simulink model "projeto_fixedstepdiscrete"  (R2015a)
settings: Solver=FixedStepDiscrete  SolverMode=SingleTasking  StartTime=0.0  StopTime=inf  RelTol=1e-3
libraries: dsparch4 x17, dspvision x14, commchan3 x1, dspsnks4 x1
settings Model: SimulationMode=accelerator  Creator=aluno  LastModifiedBy=aluno
settings DataIOCC: SaveOutput=off  SignalLogging=off  SaveTime=off
settings DebuggingCC: AlgebraicLoopMsg=error  SingleTaskRateTransMsg=error

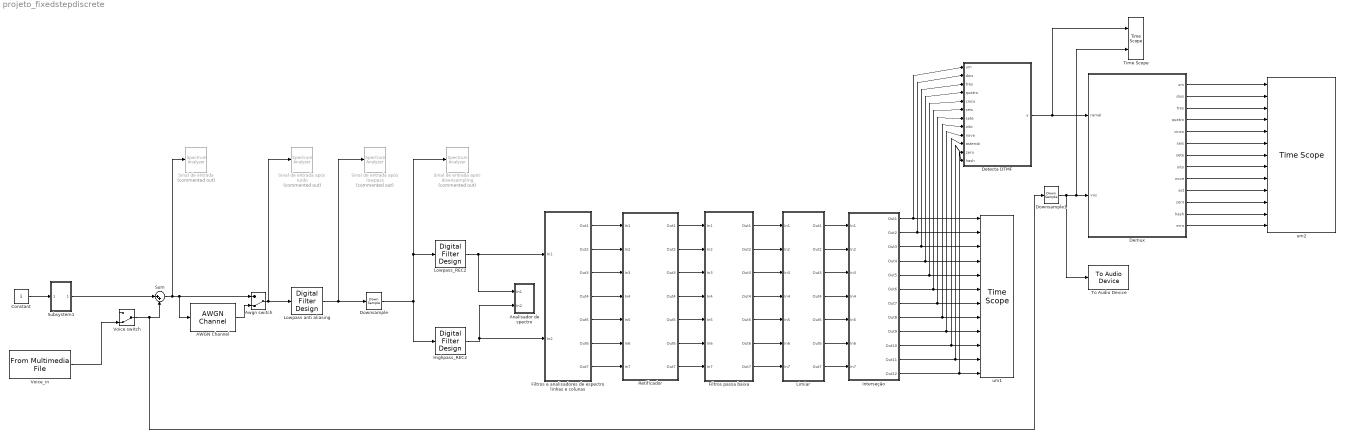
== system projeto_fixedstepdiscrete ==
  AWGN Channel : commchan3/AWGN Channel  InputProcessing=Columns as channels (frame based)  seed=67  noiseMode="Signal to noise ratio  (SNR)"  EbNodB=30  EsNodB=10  SNRdB=5  bitsPerSym=1  Ps=1  Tsym=1  variance=1
  Analisador de spectro : Subsystem
  Awgn switch : ManualSwitch  CurrentSetting=0
  Constant : Constant
  Demux : MATLAB Function  TreatAsAtomicUnit=on
  Detecta DTMF : MATLAB Function  TreatAsAtomicUnit=on
  Downsample : DownSample  N=11  RateOptions=Allow multirate processing
  Downsample1 : DownSample  N=11  RateOptions=Allow multirate processing
  Filtros e analisadores de espectro linhas e colunas : Subsystem
  Filtros passa baixa : Subsystem
  "Highpass_REC2 " : dsparch4/Digital Filter Design  mwdsp_browser_bugfix_var=off
  Interseção : Subsystem
  Limiar : Subsystem
  Lowpass anti aliasing : dsparch4/Digital Filter Design  mwdsp_browser_bugfix_var=off
  Lowpass_REC2 : dsparch4/Digital Filter Design  mwdsp_browser_bugfix_var=off
  Retificador : Subsystem
  "Sinal de entrada " : SpectrumAnalyzer  Commented=on
  "Sinal de entrada após downsampling " : SpectrumAnalyzer  Commented=on
  "Sinal de entrada após lowpass " : SpectrumAnalyzer  Commented=on
  "Sinal de entrada após ruído " : SpectrumAnalyzer  Commented=on
  Subsystem1 : Subsystem
  Sum : Sum  Inputs=|++
  Time Scope : TimeScope  DefaultConfigurationName=spbscopes.TimeScopeBlockCfg  NumInputPorts=2
  To Audio Device : dspsnks4/To Audio Device  deviceName=Default  inheritSampleRate=on  sampleRate=44100  deviceDatatype=Determine from input data type  autoBufferSize=on  bufferSize=4096  queueDuration=1.0  defaultOutputChannelMapping=on  outputChannelMapping=1:2  outputNumUnderrunSamples=off
  Voice switch : ManualSwitch  CurrentSetting=0
  "Voice_in " : dspvision/From Multimedia File  inputFilename=./Projeto_Final_PSD/Voice/voice.wav  loop=on  numPlays=inf  outputStreams=Audio only  videoDataType=single  audioDataType=double  inheritSampleTime=on  userDefinedSampleTime=1/30  noAudioOutput=off  isIntensityVideo=off  fourcc=RGB  colorVideoFormat=Separate color signals  outputEOF=off  dataOrg=Column-major  audioFrameSize=spc  computeAudioFrameSize=off  outSamplingMode=Sample based
  um1 : TimeScope  DefaultConfigurationName=spbscopes.TimeScopeBlockCfg  NumInputPorts=12
  um2 : TimeScope  DefaultConfigurationName=spbscopes.TimeScopeBlockCfg  NumInputPorts=13
  wires:
  "Voice_in "/1 -> Voice switch/2
  AWGN Channel/1 -> Awgn switch/2
  Awgn switch/1 -> Lowpass anti aliasing/1, "Sinal de entrada após ruído "/1
  Sum/1 -> "Sinal de entrada "/1, Awgn switch/1, AWGN Channel/1
  Lowpass_REC2/1 -> Analisador de spectro/1(In1), Filtros e analisadores de espectro linhas e colunas/1(In1)
  "Highpass_REC2 "/1 -> Analisador de spectro/2(In2), Filtros e analisadores de espectro linhas e colunas/2(In2)
  Downsample/1 -> "Highpass_REC2 "/1, Lowpass_REC2/1, "Sinal de entrada após downsampling "/1
  Filtros e analisadores de espectro linhas e colunas/1(Out1) -> Retificador/1(In1)
  Filtros e analisadores de espectro linhas e colunas/2(Out2) -> Retificador/2(In2)
  Filtros e analisadores de espectro linhas e colunas/3(Out3) -> Retificador/3(In3)
  Filtros e analisadores de espectro linhas e colunas/4(Out4) -> Retificador/4(In4)
  Filtros e analisadores de espectro linhas e colunas/5(Out5) -> Retificador/5(In5)
  Filtros e analisadores de espectro linhas e colunas/6(Out6) -> Retificador/6(In6)
  Filtros e analisadores de espectro linhas e colunas/7(Out7) -> Retificador/7(In7)
  Constant/1 -> Subsystem1/1(In1)
  Subsystem1/1(Out1) -> Sum/1
  Lowpass anti aliasing/1 -> Downsample/1, "Sinal de entrada após lowpass "/1
  Retificador/1(Out1) -> Filtros passa baixa/1(In1)
  Retificador/2(Out2) -> Filtros passa baixa/2(In2)
  Retificador/3(Out3) -> Filtros passa baixa/3(In3)
  Retificador/4(Out4) -> Filtros passa baixa/4(In4)
  Retificador/5(Out5) -> Filtros passa baixa/5(In5)
  Retificador/6(Out6) -> Filtros passa baixa/6(In6)
  Retificador/7(Out7) -> Filtros passa baixa/7(In7)
  Filtros passa baixa/1(Out1) -> Limiar/1(In1)
  Filtros passa baixa/2(Out2) -> Limiar/2(In2)
  Filtros passa baixa/3(Out3) -> Limiar/3(In3)
  Filtros passa baixa/4(Out4) -> Limiar/4(In4)
  Filtros passa baixa/5(Out5) -> Limiar/5(In5)
  Filtros passa baixa/6(Out6) -> Limiar/6(In6)
  Filtros passa baixa/7(Out7) -> Limiar/7(In7)
  Limiar/1(Out1) -> Interseção/1(In1)
  Limiar/2(Out2) -> Interseção/2(In2)
  Limiar/3(Out3) -> Interseção/3(In3)
  Limiar/4(Out4) -> Interseção/4(In4)
  Limiar/5(Out5) -> Interseção/5(In5)
  Limiar/6(Out6) -> Interseção/6(In6)
  Limiar/7(Out7) -> Interseção/7(In7)
  Interseção/1(Out1) -> Detecta DTMF/1(um), um1/1
  Interseção/2(Out2) -> Detecta DTMF/2(dois), um1/2
  Interseção/3(Out3) -> Detecta DTMF/3(tres), um1/3
  Interseção/5(Out5) -> um1/5, Detecta DTMF/5(cinco)
  Interseção/6(Out6) -> um1/6, Detecta DTMF/6(seis)
  Interseção/7(Out7) -> Detecta DTMF/7(sete), um1/7
  Interseção/8(Out8) -> Detecta DTMF/8(oito), um1/8
  Interseção/9(Out9) -> Detecta DTMF/9(nove), um1/9
  Interseção/10(Out10) -> Detecta DTMF/10(asterisk), um1/10
  Interseção/11(Out11) -> Detecta DTMF/11(zero), um1/11
  Interseção/12(Out12) -> Detecta DTMF/12(hash), um1/12
  Interseção/4(Out4) -> Detecta DTMF/4(quatro), um1/4
  Demux/1(um) -> um2/1
  Demux/2(dois) -> um2/2
  Demux/3(tres) -> um2/3
  Demux/4(quatro) -> um2/4
  Demux/5(cinco) -> um2/5
  Demux/6(seis) -> um2/6
  Demux/7(sete) -> um2/7
  Demux/8(oito) -> um2/8
  Demux/9(nove) -> um2/9
  Demux/10(ast) -> um2/10
  Demux/11(zero) -> um2/11
  Demux/12(hash) -> um2/12
  Voice switch/1 -> Sum/2, Downsample1/1
  Demux/13(erro) -> um2/13
  Detecta DTMF/1(y) -> Demux/1(ramal), Time Scope/1
  Downsample1/1 -> To Audio Device/1, Time Scope/2, Demux/2(voz)

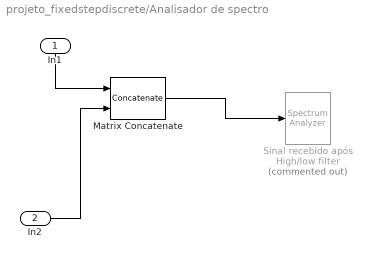
== system projeto_fixedstepdiscrete/Analisador de spectro ==
  In1 : Inport
  In2 : Inport  Port=2
  Matrix Concatenate : Concatenate  Mode=Multidimensional array  ConcatenateDimension=2
  Sinal recebido após High/low filter : SpectrumAnalyzer  Commented=on
  wires:
  In1/1 -> Matrix Concatenate/1
  In2/1 -> Matrix Concatenate/2
  Matrix Concatenate/1 -> Sinal recebido após High/low filter/1

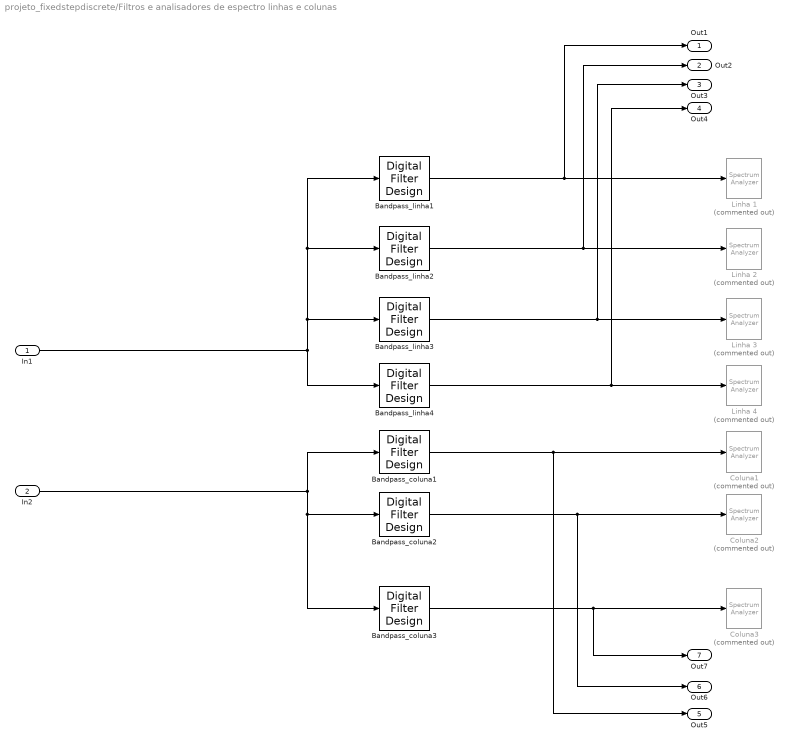
== system projeto_fixedstepdiscrete/Filtros e analisadores de espectro linhas e colunas ==
  In1 : Inport
  In2 : Inport  Port=2
  Bandpass_coluna1 : dsparch4/Digital Filter Design  mwdsp_browser_bugfix_var=off
  Bandpass_coluna2 : dsparch4/Digital Filter Design  mwdsp_browser_bugfix_var=off
  Bandpass_coluna3 : dsparch4/Digital Filter Design  mwdsp_browser_bugfix_var=off
  Bandpass_linha{1..4} (4 alike) : dsparch4/Digital Filter Design  mwdsp_browser_bugfix_var=off
  "Coluna1 " : SpectrumAnalyzer  Commented=on
  "Coluna2 " : SpectrumAnalyzer  Commented=on
  Coluna3 : SpectrumAnalyzer  Commented=on
  Linha {1..4} (4 alike) : SpectrumAnalyzer  Commented=on
  Out1 : Outport
  Out2 : Outport  Port=2
  Out3 : Outport  Port=3
  Out4 : Outport  Port=4
  Out5 : Outport  Port=5
  Out6 : Outport  Port=6
  Out7 : Outport  Port=7
  wires:
  In1/1 -> Bandpass_linha4/1, Bandpass_linha3/1, Bandpass_linha2/1, Bandpass_linha1/1
  In2/1 -> Bandpass_coluna1/1, Bandpass_coluna2/1, Bandpass_coluna3/1
  Bandpass_linha1/1 -> Out1/1, Linha 1/1
  Bandpass_linha4/1 -> Out4/1, Linha 4/1
  Bandpass_linha2/1 -> Out2/1, Linha 2/1
  Bandpass_coluna3/1 -> Out7/1, Coluna3/1
  Bandpass_coluna2/1 -> Out6/1, "Coluna2 "/1
  Bandpass_linha3/1 -> Out3/1, Linha 3/1
  Bandpass_coluna1/1 -> Out5/1, "Coluna1 "/1

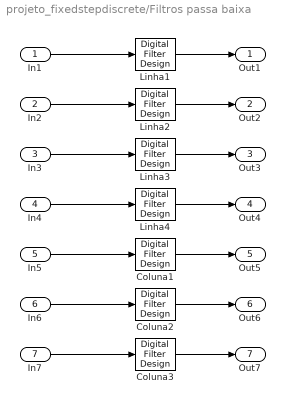
== system projeto_fixedstepdiscrete/Filtros passa baixa ==
  In1 : Inport
  In2 : Inport  Port=2
  In3 : Inport  Port=3
  In4 : Inport  Port=4
  In5 : Inport  Port=5
  In6 : Inport  Port=6
  In7 : Inport  Port=7
  Coluna1 : dsparch4/Digital Filter Design  mwdsp_browser_bugfix_var=off
  Coluna2 : dsparch4/Digital Filter Design  mwdsp_browser_bugfix_var=off
  Coluna3 : dsparch4/Digital Filter Design  mwdsp_browser_bugfix_var=off
  Linha{1..4} (4 alike) : dsparch4/Digital Filter Design  mwdsp_browser_bugfix_var=off
  Out1 : Outport
  Out2 : Outport  Port=2
  Out3 : Outport  Port=3
  Out4 : Outport  Port=4
  Out5 : Outport  Port=5
  Out6 : Outport  Port=6
  Out7 : Outport  Port=7
  wires:
  Linha2/1 -> Out2/1
  Coluna3/1 -> Out7/1
  Linha4/1 -> Out4/1
  Linha3/1 -> Out3/1
  In1/1 -> Linha1/1
  In2/1 -> Linha2/1
  In3/1 -> Linha3/1
  In4/1 -> Linha4/1
  In5/1 -> Coluna1/1
  In6/1 -> Coluna2/1
  In7/1 -> Coluna3/1
  Linha1/1 -> Out1/1
  Coluna1/1 -> Out5/1
  Coluna2/1 -> Out6/1

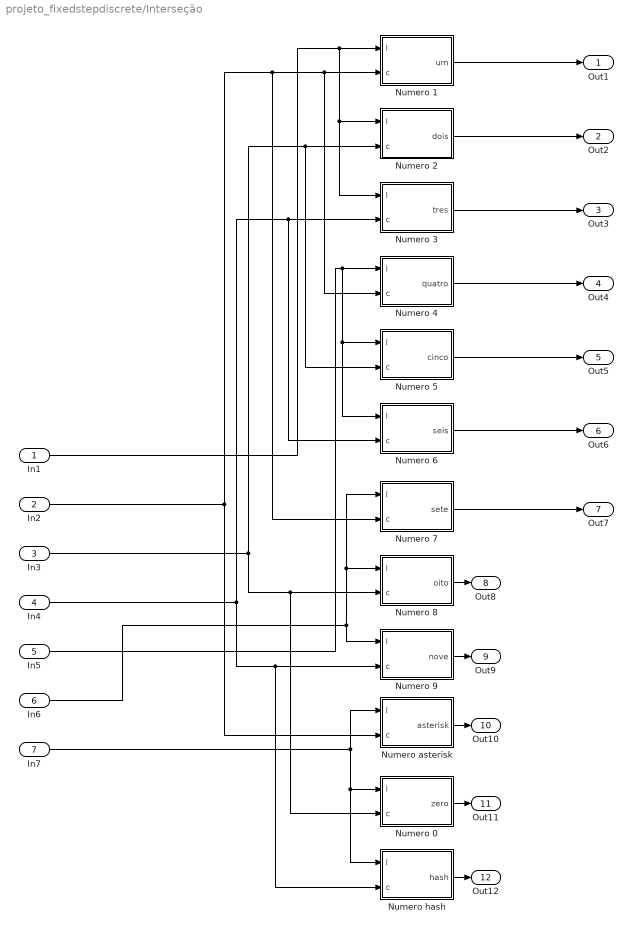
== system projeto_fixedstepdiscrete/Interseção ==
  In1 : Inport
  In2 : Inport  Port=2
  In3 : Inport  Port=3
  In4 : Inport  Port=4
  In5 : Inport  Port=5
  In6 : Inport  Port=6
  In7 : Inport  Port=7
  Numero 0 : MATLAB Function  TreatAsAtomicUnit=on
  Numero 1 : MATLAB Function  TreatAsAtomicUnit=on
  Numero 2 : MATLAB Function  TreatAsAtomicUnit=on
  Numero 3 : MATLAB Function  TreatAsAtomicUnit=on
  Numero 4 : MATLAB Function  TreatAsAtomicUnit=on
  Numero 5 : MATLAB Function  TreatAsAtomicUnit=on
  Numero 6 : MATLAB Function  TreatAsAtomicUnit=on
  Numero 7 : MATLAB Function  TreatAsAtomicUnit=on
  Numero 8 : MATLAB Function  TreatAsAtomicUnit=on
  Numero 9 : MATLAB Function  TreatAsAtomicUnit=on
  Numero asterisk : MATLAB Function  TreatAsAtomicUnit=on
  Numero hash : MATLAB Function  TreatAsAtomicUnit=on
  Out1 : Outport
  Out2 : Outport  Port=2
  Out3 : Outport  Port=3
  Out4 : Outport  Port=4
  Out5 : Outport  Port=5
  Out6 : Outport  Port=6
  Out7 : Outport  Port=7
  Out8 : Outport  Port=8
  Out9 : Outport  Port=9
  Out10 : Outport  Port=10
  Out11 : Outport  Port=11
  Out12 : Outport  Port=12
  wires:
  Numero 4/1(quatro) -> Out4/1
  Numero 9/1(nove) -> Out9/1
  In5/1 -> Numero 4/1(l), Numero 6/1(l), Numero 5/1(l)
  Numero 2/1(dois) -> Out2/1
  In1/1 -> Numero 3/1(l), Numero 2/1(l), Numero 1/1(l)
  Numero 5/1(cinco) -> Out5/1
  Numero 8/1(oito) -> Out8/1
  In3/1 -> Numero 0/2(c), Numero 8/2(c), Numero 5/2(c), Numero 2/2(c)
  In7/1 -> Numero hash/1(l), Numero 0/1(l), Numero asterisk/1(l)
  Numero 0/1(zero) -> Out11/1
  Numero hash/1(hash) -> Out12/1
  In6/1 -> Numero 7/1(l), Numero 8/1(l), Numero 9/1(l)
  Numero 7/1(sete) -> Out7/1
  Numero 6/1(seis) -> Out6/1
  Numero 3/1(tres) -> Out3/1
  In4/1 -> Numero hash/2(c), Numero 9/2(c), Numero 6/2(c), Numero 3/2(c)
  Numero asterisk/1(asterisk) -> Out10/1
  In2/1 -> Numero asterisk/2(c), Numero 7/2(c), Numero 4/2(c), Numero 1/2(c)
  Numero 1/1(um) -> Out1/1

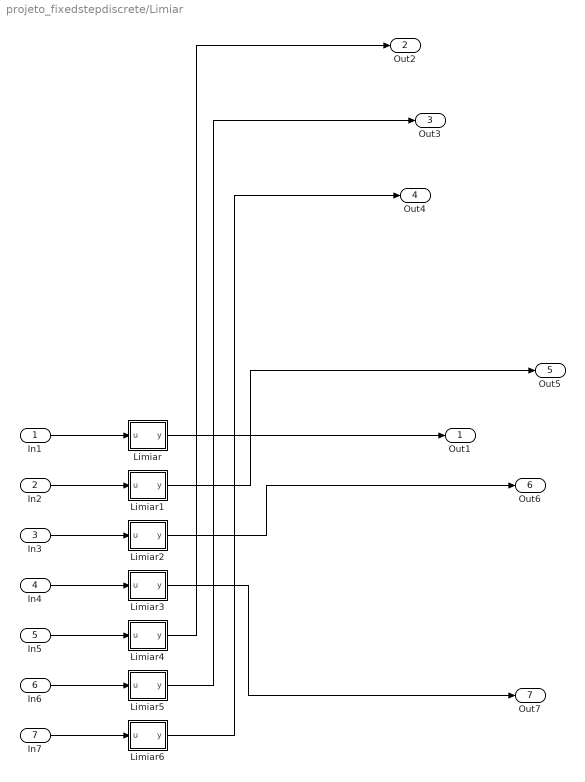
== system projeto_fixedstepdiscrete/Limiar ==
  In1 : Inport
  In2 : Inport  Port=2
  In3 : Inport  Port=3
  In4 : Inport  Port=4
  In5 : Inport  Port=5
  In6 : Inport  Port=6
  In7 : Inport  Port=7
  Limiar : MATLAB Function  TreatAsAtomicUnit=on
  Limiar1 : MATLAB Function  TreatAsAtomicUnit=on
  Limiar2 : MATLAB Function  TreatAsAtomicUnit=on
  Limiar3 : MATLAB Function  TreatAsAtomicUnit=on
  Limiar4 : MATLAB Function  TreatAsAtomicUnit=on
  Limiar5 : MATLAB Function  TreatAsAtomicUnit=on
  Limiar6 : MATLAB Function  TreatAsAtomicUnit=on
  Out1 : Outport
  Out2 : Outport  Port=2
  Out3 : Outport  Port=3
  Out4 : Outport  Port=4
  Out5 : Outport  Port=5
  Out6 : Outport  Port=6
  Out7 : Outport  Port=7
  wires:
  Limiar2/1(y) -> Out6/1
  Limiar4/1(y) -> Out2/1
  Limiar/1(y) -> Out1/1
  Limiar1/1(y) -> Out5/1
  In1/1 -> Limiar/1(u)
  In7/1 -> Limiar6/1(u)
  In6/1 -> Limiar5/1(u)
  In5/1 -> Limiar4/1(u)
  In3/1 -> Limiar2/1(u)
  In4/1 -> Limiar3/1(u)
  In2/1 -> Limiar1/1(u)
  Limiar6/1(y) -> Out4/1
  Limiar3/1(y) -> Out7/1
  Limiar5/1(y) -> Out3/1

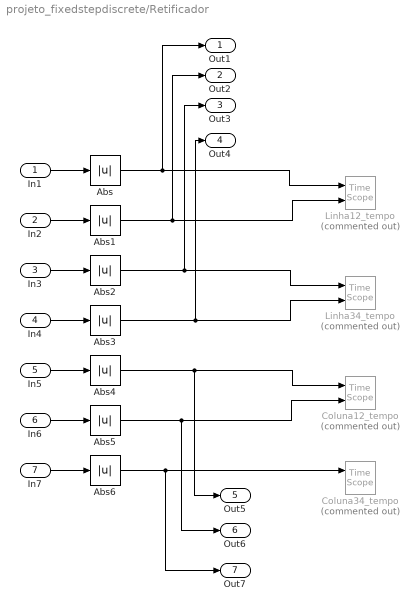
== system projeto_fixedstepdiscrete/Retificador ==
  In1 : Inport
  In2 : Inport  Port=2
  In3 : Inport  Port=3
  In4 : Inport  Port=4
  In5 : Inport  Port=5
  In6 : Inport  Port=6
  In7 : Inport  Port=7
  Abs{,1..6} (7 alike) : Abs
  Coluna12_tempo : TimeScope  Commented=on  DefaultConfigurationName=spbscopes.TimeScopeBlockCfg  NumInputPorts=2
  Coluna34_tempo : TimeScope  Commented=on  DefaultConfigurationName=spbscopes.TimeScopeBlockCfg  NumInputPorts=2
  "Linha12_tempo " : TimeScope  Commented=on  DefaultConfigurationName=spbscopes.TimeScopeBlockCfg  NumInputPorts=2
  Linha34_tempo : TimeScope  Commented=on  DefaultConfigurationName=spbscopes.TimeScopeBlockCfg  NumInputPorts=2
  Out1 : Outport
  Out2 : Outport  Port=2
  Out3 : Outport  Port=3
  Out4 : Outport  Port=4
  Out5 : Outport  Port=5
  Out6 : Outport  Port=6
  Out7 : Outport  Port=7
  wires:
  Abs6/1 -> Out7/1, Coluna34_tempo/1
  Abs5/1 -> Coluna12_tempo/2, Out6/1
  Abs4/1 -> Out5/1, Coluna12_tempo/1
  Abs2/1 -> Out3/1, Linha34_tempo/1
  Abs3/1 -> Out4/1, Linha34_tempo/2
  In6/1 -> Abs5/1
  In3/1 -> Abs2/1
  In4/1 -> Abs3/1
  In2/1 -> Abs1/1
  Abs1/1 -> Out2/1, "Linha12_tempo "/2
  In7/1 -> Abs6/1
  Abs/1 -> Out1/1, "Linha12_tempo "/1
  In5/1 -> Abs4/1
  In1/1 -> Abs/1

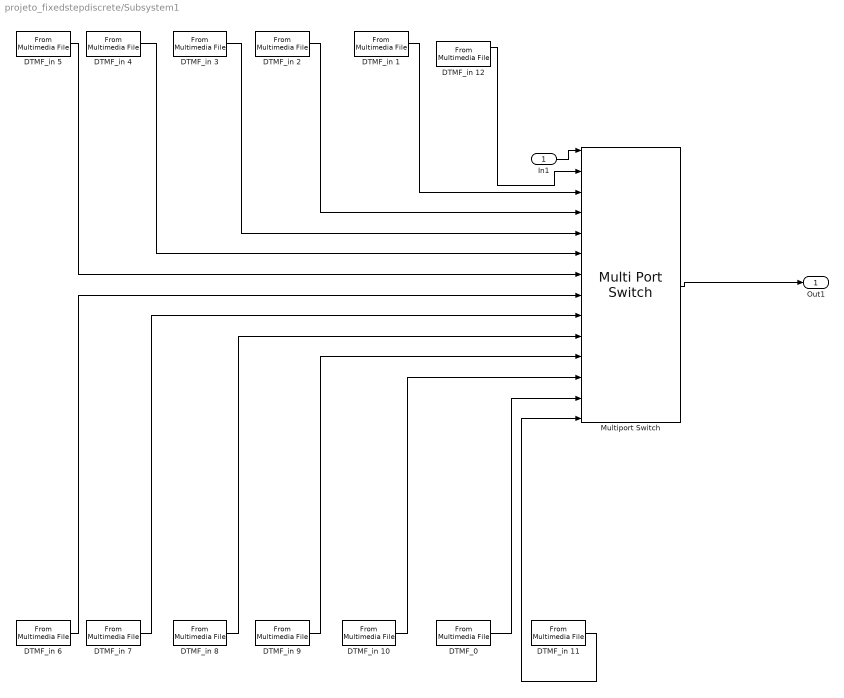
== system projeto_fixedstepdiscrete/Subsystem1 ==
  In1 : Inport
  "DTMF_0 " : dspvision/From Multimedia File  inputFilename=./Projeto_Final_PSD/Audios DTMF com Pausa/0-DTMF.wav  loop=on  numPlays=inf  outputStreams=Audio only  videoDataType=single  audioDataType=double  inheritSampleTime=on  userDefinedSampleTime=1/30  noAudioOutput=off  isIntensityVideo=off  fourcc=RGB  colorVideoFormat=Separate color signals  outputEOF=off  dataOrg=Column-major  audioFrameSize=spc  computeAudioFrameSize=off  outSamplingMode=Sample based
  DTMF_in 1 : dspvision/From Multimedia File  inputFilename=./Projeto_Final_PSD/Audios DTMF com Pausa/1-DTMF.wav  loop=on  numPlays=inf  outputStreams=Audio only  videoDataType=single  audioDataType=double  inheritSampleTime=on  userDefinedSampleTime=1/30  noAudioOutput=off  isIntensityVideo=off  fourcc=RGB  colorVideoFormat=Separate color signals  outputEOF=off  dataOrg=Column-major  audioFrameSize=spc  computeAudioFrameSize=off  outSamplingMode=Sample based
  DTMF_in 10 : dspvision/From Multimedia File  inputFilename=./Projeto_Final_PSD/Audios DTMF com Pausa/Asterisk.wav  loop=on  numPlays=inf  outputStreams=Audio only  videoDataType=single  audioDataType=double  inheritSampleTime=on  userDefinedSampleTime=1/30  noAudioOutput=off  isIntensityVideo=off  fourcc=RGB  colorVideoFormat=Separate color signals  outputEOF=off  dataOrg=Column-major  audioFrameSize=spc  computeAudioFrameSize=off  outSamplingMode=Sample based
  DTMF_in 11 : dspvision/From Multimedia File  inputFilename=./Projeto_Final_PSD/Audios DTMF com Pausa/Hash-DTMF.wav  loop=on  numPlays=inf  outputStreams=Audio only  videoDataType=single  audioDataType=double  inheritSampleTime=on  userDefinedSampleTime=1/30  noAudioOutput=off  isIntensityVideo=off  fourcc=RGB  colorVideoFormat=Separate color signals  outputEOF=off  dataOrg=Column-major  audioFrameSize=spc  computeAudioFrameSize=off  outSamplingMode=Sample based
  DTMF_in 12 : dspvision/From Multimedia File  inputFilename=./Projeto_Final_PSD/Audios DTMF com Pausa/Sequencia-DTMF.wav  loop=on  numPlays=inf  outputStreams=Audio only  videoDataType=single  audioDataType=double  inheritSampleTime=on  userDefinedSampleTime=1/30  noAudioOutput=off  isIntensityVideo=off  fourcc=RGB  colorVideoFormat=Separate color signals  outputEOF=on  dataOrg=Column-major  audioFrameSize=spc  computeAudioFrameSize=off  outSamplingMode=Sample based
  DTMF_in 2 : dspvision/From Multimedia File  inputFilename=./Projeto_Final_PSD/Audios DTMF com Pausa/2-DTMF.wav  loop=on  numPlays=inf  outputStreams=Audio only  videoDataType=single  audioDataType=double  inheritSampleTime=on  userDefinedSampleTime=1/30  noAudioOutput=off  isIntensityVideo=off  fourcc=RGB  colorVideoFormat=Separate color signals  outputEOF=off  dataOrg=Column-major  audioFrameSize=spc  computeAudioFrameSize=off  outSamplingMode=Sample based
  DTMF_in 3 : dspvision/From Multimedia File  inputFilename=./Projeto_Final_PSD/Audios DTMF com Pausa/3-DTMF.wav  loop=on  numPlays=inf  outputStreams=Audio only  videoDataType=single  audioDataType=double  inheritSampleTime=on  userDefinedSampleTime=1/30  noAudioOutput=off  isIntensityVideo=off  fourcc=RGB  colorVideoFormat=Separate color signals  outputEOF=off  dataOrg=Column-major  audioFrameSize=spc  computeAudioFrameSize=off  outSamplingMode=Sample based
  DTMF_in 4 : dspvision/From Multimedia File  inputFilename=./Projeto_Final_PSD/Audios DTMF com Pausa/4-DTMF.wav  loop=on  numPlays=inf  outputStreams=Audio only  videoDataType=single  audioDataType=double  inheritSampleTime=on  userDefinedSampleTime=1/30  noAudioOutput=off  isIntensityVideo=off  fourcc=RGB  colorVideoFormat=Separate color signals  outputEOF=off  dataOrg=Column-major  audioFrameSize=spc  computeAudioFrameSize=off  outSamplingMode=Sample based
  DTMF_in 5 : dspvision/From Multimedia File  inputFilename=./Projeto_Final_PSD/Audios DTMF com Pausa/5-DTMF.wav  loop=on  numPlays=inf  outputStreams=Audio only  videoDataType=single  audioDataType=double  inheritSampleTime=on  userDefinedSampleTime=1/30  noAudioOutput=off  isIntensityVideo=off  fourcc=RGB  colorVideoFormat=Separate color signals  outputEOF=off  dataOrg=Column-major  audioFrameSize=spc  computeAudioFrameSize=off  outSamplingMode=Sample based
  DTMF_in 6 : dspvision/From Multimedia File  inputFilename=./Projeto_Final_PSD/Audios DTMF com Pausa/6-DTMF.wav  loop=on  numPlays=inf  outputStreams=Audio only  videoDataType=single  audioDataType=double  inheritSampleTime=on  userDefinedSampleTime=1/30  noAudioOutput=off  isIntensityVideo=off  fourcc=RGB  colorVideoFormat=Separate color signals  outputEOF=off  dataOrg=Column-major  audioFrameSize=spc  computeAudioFrameSize=off  outSamplingMode=Sample based
  DTMF_in 7 : dspvision/From Multimedia File  inputFilename=./Projeto_Final_PSD/Audios DTMF com Pausa/7-DTMF.wav  loop=on  numPlays=inf  outputStreams=Audio only  videoDataType=single  audioDataType=double  inheritSampleTime=on  userDefinedSampleTime=1/30  noAudioOutput=off  isIntensityVideo=off  fourcc=RGB  colorVideoFormat=Separate color signals  outputEOF=off  dataOrg=Column-major  audioFrameSize=spc  computeAudioFrameSize=off  outSamplingMode=Sample based
  DTMF_in 8 : dspvision/From Multimedia File  inputFilename=./Projeto_Final_PSD/Audios DTMF com Pausa/8-DTMF.wav  loop=on  numPlays=inf  outputStreams=Audio only  videoDataType=single  audioDataType=double  inheritSampleTime=on  userDefinedSampleTime=1/30  noAudioOutput=off  isIntensityVideo=off  fourcc=RGB  colorVideoFormat=Separate color signals  outputEOF=off  dataOrg=Column-major  audioFrameSize=spc  computeAudioFrameSize=off  outSamplingMode=Sample based
  DTMF_in 9 : dspvision/From Multimedia File  inputFilename=./Projeto_Final_PSD/Audios DTMF com Pausa/9-DTMF.wav  loop=on  numPlays=inf  outputStreams=Audio only  videoDataType=single  audioDataType=double  inheritSampleTime=on  userDefinedSampleTime=1/30  noAudioOutput=off  isIntensityVideo=off  fourcc=RGB  colorVideoFormat=Separate color signals  outputEOF=off  dataOrg=Column-major  audioFrameSize=spc  computeAudioFrameSize=off  outSamplingMode=Sample based
  Multiport Switch : MultiPortSwitch  DataPortOrder=Specify indices  Inputs=12  DataPortIndices={0,1,2,3,4,5,6,7,8,9,10,11,12}
  Out1 : Outport
  wires:
  DTMF_in 7/1 -> Multiport Switch/9
  Multiport Switch/1 -> Out1/1
  DTMF_in 3/1 -> Multiport Switch/5
  DTMF_in 5/1 -> Multiport Switch/7
  DTMF_in 8/1 -> Multiport Switch/10
  In1/1 -> Multiport Switch/1
  DTMF_in 1/1 -> Multiport Switch/3
  DTMF_in 4/1 -> Multiport Switch/6
  DTMF_in 9/1 -> Multiport Switch/11
  DTMF_in 10/1 -> Multiport Switch/12
  DTMF_in 2/1 -> Multiport Switch/4
  DTMF_in 6/1 -> Multiport Switch/8
  DTMF_in 12/1 -> Multiport Switch/2
  "DTMF_0 "/1 -> Multiport Switch/13
  DTMF_in 11/1 -> Multiport Switch/14

== matlab function projeto_fixedstepdiscrete/Interseção/Numero 2 ==
  data: l input; dois output; c input

function dois = fcn(l,c)
%#codegen

if (l == 1 && c == 1) 
    u = 1;
else 
    u = 0;
end


dois = u;

== matlab function projeto_fixedstepdiscrete/Limiar/Limiar ==
  data: u input; y output

function y = fcn(u)
%#codegen

u = (u>0.2);

y = u;

== matlab function projeto_fixedstepdiscrete/Interseção/Numero 1 ==
  data: l input; um output; c input

function um = fcn(l,c)
%#codegen

if (l == 1 && c == 1) 
    u = 1;
else 
    u = 0;
end


um = u;

== matlab function projeto_fixedstepdiscrete/Limiar/Limiar1 ==
  data: u input; y output

function y = fcn(u)
%#codegen

u = (u>0.2);

y = u;

== matlab function projeto_fixedstepdiscrete/Limiar/Limiar2 ==
  data: u input; y output

function y = fcn(u)
%#codegen

u = (u>0.2);

y = u;

== matlab function projeto_fixedstepdiscrete/Limiar/Limiar3 ==
  data: u input; y output

function y = fcn(u)
%#codegen

u = (u>0.2);

y = u;

== matlab function projeto_fixedstepdiscrete/Limiar/Limiar4 ==
  data: u input; y output

function y = fcn(u)
%#codegen

u = (u>0.2);

y = u;

== matlab function projeto_fixedstepdiscrete/Limiar/Limiar5 ==
  data: u input; y output

function y = fcn(u)
%#codegen

u = (u>0.2);

y = u;

== matlab function projeto_fixedstepdiscrete/Limiar/Limiar6 ==
  data: u input; y output

function y = fcn(u)
%#codegen

u = (u>0.2);

y = u;

== matlab function projeto_fixedstepdiscrete/Interseção/Numero 3 ==
  data: l input; tres output; c input

function tres = fcn(l,c)
%#codegen

if (l == 1 && c == 1) 
    u = 1;
else 
    u = 0;
end


tres = u;

== matlab function projeto_fixedstepdiscrete/Interseção/Numero 4 ==
  data: l input; quatro output; c input

function quatro = fcn(l,c)
%#codegen

if (l == 1 && c == 1) 
    u = 1;
else 
    u = 0;
end


quatro = u;

== matlab function projeto_fixedstepdiscrete/Interseção/Numero 5 ==
  data: l input; cinco output; c input

function cinco = fcn(l,c)
%#codegen

if (l == 1 && c == 1) 
    u = 1;
else 
    u = 0;
end


cinco = u;

== matlab function projeto_fixedstepdiscrete/Interseção/Numero 6 ==
  data: l input; seis output; c input

function seis = fcn(l,c)
%#codegen

if (l == 1 && c == 1) 
    u = 1;
else 
    u = 0;
end


seis = u;

== matlab function projeto_fixedstepdiscrete/Interseção/Numero 7 ==
  data: l input; sete output; c input

function sete = fcn(l,c)
%#codegen

if (l == 1 && c == 1) 
    u = 1;
else 
    u = 0;
end


sete = u;

== matlab function projeto_fixedstepdiscrete/Interseção/Numero 8 ==
  data: l input; oito output; c input

function oito = fcn(l,c)
%#codegen

if (l == 1 && c == 1) 
    u = 1;
else 
    u = 0;
end


oito = u;

== matlab function projeto_fixedstepdiscrete/Interseção/Numero 9 ==
  data: l input; nove output; c input

function nove = fcn(l,c)
%#codegen

if (l == 1 && c == 1) 
    u = 1;
else 
    u = 0;
end


nove = u;

== matlab function projeto_fixedstepdiscrete/Interseção/Numero asterisk ==
  data: l input; asterisk output; c input

function asterisk = fcn(l,c)
%#codegen

if (l == 1 && c == 1) 
    u = 1;
else 
    u = 0;
end


asterisk = u;

== matlab function projeto_fixedstepdiscrete/Interseção/Numero 0 ==
  data: l input; zero output; c input

function zero = fcn(l,c)
%#codegen

if (l == 1 && c == 1) 
    u = 1;
else 
    u = 0;
end


zero = u;

== matlab function projeto_fixedstepdiscrete/Interseção/Numero hash ==
  data: l input; hash output; c input

function hash = fcn(l,c)
%#codegen

if (l == 1 && c == 1) 
    u = 1;
else 
    u = 0;
end


hash = u;

== matlab function projeto_fixedstepdiscrete/Detecta DTMF ==
  data: um input; y output; dois input; tres input; quatro input; cinco input; seis input; sete input; oito input; nove input; asterisk input; zero input; hash input
function y = fcn(um,dois,tres,quatro,cinco,seis,sete,oito,nove,asterisk,zero,hash)
%#codegen
u = 14;
persistent c_um c_dois c_tres c_quatro c_cinco c_seis c_sete c_oito c_nove c_asterisk c_zero c_hash;

if isempty(c_um)
    c_um=0; c_dois=0; c_tres=0; c_quatro=0; c_cinco=0; c_seis=0; c_sete=0; c_oito=0; c_nove=0; c_asterisk=0; c_zero=0; c_hash=0;
end

p_um=0; p_dois=0; p_tres=0; p_quatro=0; p_cinco=0; p_seis=0; p_sete=0; p_oito=0; p_nove=0; p_asterisk=0; p_zero=0; p_hash=0;

%% Bloco que verifica se a amostra é 1.
if(um == 1) 
   c_um = c_um + 1;
end
if(dois == 1) 
   c_dois = c_dois + 1;
end
if(tres == 1) 
   c_tres = c_tres + 1;
end
if(quatro == 1) 
   c_quatro = c_quatro + 1;
end
if(cinco == 1) 
   c_cinco = c_cinco + 1;
end
if(seis == 1) 
   c_seis = c_seis + 1;
end
if(sete == 1) 
   c_sete = c_sete + 1;
end
if(oito == 1) 
   c_oito = c_oito + 1;
end
if(nove == 1) 
   c_nove = c_nove + 1;
end
if(asterisk == 1) 
   c_asterisk = c_asterisk + 1;
end
if(zero == 1) 
   c_zero = c_zero + 1;
end
if(hash == 1) 
   c_hash = c_hash + 1;
end

%% Bloco que verifica quantas amostras chegaram em 1.
if(c_um == 160)
    p_um = 1;
    c_um = 0;
    disp('digitou um');
end
if(c_dois == 160)
    p_dois = 1;
    c_dois = 0;
    disp('digitou dois');
end
if(c_tres == 160)
    p_tres = 1;
    c_tres = 0;
    disp('digitou tres');
end
if(c_quatro == 160)
    p_quatro = 1;
    c_quatro = 0;
    disp('digitou quatro');
end
if(c_cinco == 160)
    p_cinco = 1;
    c_cinco = 0;
    disp('digitou cinco');
end
if(c_seis == 160)
    p_seis = 1;
    c_seis = 0;
    disp('digitou seis');
end
if(c_sete == 160)
    p_sete = 1;
    c_sete = 0;
    disp('digitou sete');
end
if(c_oito == 160)
    p_oito = 1;
    c_oito = 0;
    disp('digitou oito');
end
if(c_nove == 160)
    p_nove = 1;
    c_nove = 0;
    disp('digitou nove');
end
if(c_asterisk == 160)
    p_asterisk = 1;
    c_asterisk = 0;
    disp('digitou asterisk');
end
if(c_zero == 160)
    p_zero = 1;
    c_zero = 0;
    disp('digitou zero');
end
if(c_hash == 160)
    p_hash = 1;
    c_hash = 0;
    disp('digitou hash');
end
%% Bloco que verifica quantos foram discados



if((p_um+p_dois+p_tres+p_quatro+p_cinco+p_seis+p_sete+p_oito+p_nove+p_asterisk+p_zero+p_hash) > 1)
    disp('erro');
end

if(p_um == 1)
    u = 1;
    p_um = 0;
end
if(p_dois == 1)
    u = 2;
    p_dois = 0;
end
if(p_tres == 1)
    u = 3;
    p_tres = 0;
end
if(p_quatro == 1)
    u = 4;
    p_quatro = 0;
end
if(p_cinco == 1)
    u = 5;
    p_cinco = 0;
end
if(p_seis == 1)
    u = 6;
    p_seis = 0;
end
if(p_sete == 1)
    u = 7;
    p_sete = 0;
end
if(p_oito == 1)
    u = 8;
    p_oito = 0;
end
if(p_nove == 1)
    u = 9;
    p_nove = 0;
end
if(p_asterisk == 1)
    u = 10;
    p_oito = 0;
end
if(p_zero == 1)
    u = 0;
    p_zerp = 0;
end
if(p_hash == 1)
    u = 11;
    p_hash = 0;
end


y = u;

== matlab function projeto_fixedstepdiscrete/Demux ==
  data: um output; dois output; ramal input; tres output; quatro output; cinco output; seis output; sete output; oito output; nove output; ast output; zero output; hash output; voz input; erro output
function [um,dois,tres,quatro,cinco,seis,sete,oito,nove,ast,zero,hash,erro]= fcn(ramal,voz)
%#codegen
um=0;dois=0;tres=0;quatro=0;cinco=0;seis=0;sete=0;oito=0;nove=0;ast=0;hash=0;zero=0;erro=01010;

persistent c_um c_dois c_tres c_quatro c_cinco c_seis c_sete c_oito c_nove c_ast c_zero c_hash;

if (isempty(c_um) && isempty(c_dois) && isempty(c_tres) && isempty(c_quatro) && isempty(c_cinco) && isempty(c_seis) && isempty(c_sete) &&isempty(c_oito) && isempty(c_nove) && isempty(c_ast) && isempty(c_zero) && isempty(c_hash)) 
    if (ramal == 1)
        um = voz;
        c_um = voz;
    elseif (ramal == 2)
        dois = voz;
        c_dois = voz;
    elseif (ramal == 3)
        tres = voz;
        c_tres = voz;
    elseif (ramal == 4)
        quatro = voz;
        c_quatro = voz;
    elseif (ramal == 5)
        cinco = voz;
        c_cinco = voz;
    elseif (ramal == 6)
        seis = voz;
        c_seis = voz;
    elseif (ramal == 7)
        sete = voz;
        c_sete = voz;
    elseif (ramal == 8)
        oito = voz;
        c_oito = voz;
    elseif (ramal == 9)
        nove = voz;
        c_nove = voz;
    elseif (ramal == 10)
        ast = voz;
        c_ast = voz;
    elseif (ramal == 11)
        hash = voz;
        c_hash = voz;
    elseif (ramal == 0)
        zero = voz;
        c_zero = voz;
    else 
        erro = 01010;
    end
end

if(~isempty(c_um))
    um = voz;
end
if(~isempty(c_dois))
    dois = voz;
end
if(~isempty(c_tres))
    tres = voz;
end
if(~isempty(c_quatro))
    quatro = voz;
end
if(~isempty(c_cinco))
    cinco = voz;
end
if(~isempty(c_seis))
    seis = voz;
end
if(~isempty(c_sete))
    sete = voz;
end
if(~isempty(c_oito))
    oito = voz;
end
if(~isempty(c_nove))
    nove = voz;
end
if(~isempty(c_ast))
    ast = voz;
end
if(~isempty(c_zero))
    zero = voz;
end
if(~isempty(c_hash))
    hash = voz;
end
